simulink model "DA40_Flight_Model"  (R2023a)
settings: Solver=FixedStepAuto  StartTime=DCAM.startTime  StopTime=DCAM.endTime  FixedStep=DCAM.timeStep  RelTol=1e-3
undefined symbols (not defined in the file or in its folder): DCAM, Earth, WGS84
libraries: simulink x27, slpidlib x15, simulink_extras x6, sharedtransform x4, aerolibtransform2 x4, aerolibatmos2 x3, uavalgslib x2, aerolibwind2 x1
(part 5 of 6)

== matlab function DA40_Flight_Model/Correlator Simulation/Subsystem1/Generating GPS and Satellite Measurements/Calculate Satellite Positions/MATLAB Function ==
  data: transmitTime input; satelliteID input; toe input; a_f2 input; a_f1 input; a_f0 input; T_GD input; sqrtA input; Eccentricity input; C_us input; C_uc input; satX output; satY output; satZ output; satU output; satV output; satW output; satClkCorr output; C_rs input; C_rc input; C_is input; C_ic input; M_0 input; iDOT input; i_0 input; OMEGA input; OMEGA_DOT input; delta_n input; OMEGA_0 input
function [satX,satY,satZ,satU,satV,satW,satClkCorr] = satpos(transmitTime,satelliteID,toe,a_f2,a_f1,a_f0,T_GD,sqrtA,Eccentricity,C_us,C_uc,C_rs,C_rc,C_is,C_ic,M_0,iDOT,i_0,OMEGA,OMEGA_DOT,delta_n,OMEGA_0)

%% Initialize constants ===================================================
numOfSatellites = length(satelliteID);

% GPS constatns

gpsPi          = 3.1415926535898;  % Pi used in the GPS coordinate
% system

%--- Constants for satellite position calculation -------------------------
Omegae_dot     = 7.2921151467e-5;  % Earth rotation rate, [rad/s]
GM             = 3.986005e14;      % Earth's universal
% gravitational parameter,
% [m^3/s^2]
F              = -4.442807633e-10; % Constant, [sec/(meter)^(1/2)]

%% Initialize results =====================================================
satClkCorr   = zeros(1,numOfSatellites);
satX = zeros(1,numOfSatellites);
satY = zeros(1,numOfSatellites);
satZ = zeros(1,numOfSatellites);
satU = zeros(1,numOfSatellites);
satV = zeros(1,numOfSatellites);
satW = zeros(1,numOfSatellites);

%% Process each satellite =================================================

for satNr = 1 : numOfSatellites

    %% Find initial satellite clock correction --------------------------------

    %--- Find time difference ---------------------------------------------
    dt = check_t(transmitTime(satNr) - toe(satNr));

    %--- Calculate clock correction ---------------------------------------
    satClkCorr(satNr) = (a_f2(satNr) * dt + a_f1(satNr)) * dt + ...
        a_f0(satNr) - ...
        T_GD(satNr);
    time = transmitTime(satNr) - satClkCorr(satNr);

    %% Find satellite's position ----------------------------------------------

    % Restore semi-major axis
    a   = sqrtA(satNr)*sqrtA(satNr);

    % Time correction
    tk  = check_t(time - toe(satNr));

    % Initial mean motion
    n0  = sqrt(GM/a^3);
    % Mean motion
    n   = n0 + delta_n(satNr);

    % Mean anomaly
    M   = M_0(satNr) + n*tk;
    % Reduce mean anomaly to between 0 and 360 deg
    M   = rem(M + 2*gpsPi, 2*gpsPi);

    % Initial guess of eccentric anomaly
    E   = M;

    %--- Iteratively compute eccentric anomaly ----------------------------
    for ii = 1:10
        E_old   = E;
        E       = M + Eccentricity(satNr) * sin(E);
        dE      = rem(E - E_old, 2*gpsPi);

        if abs(dE) < 1.e-12
            % Necessary precision is reached, exit from the loop
            break;
        end
    end

    % Reduce eccentric anomaly to between 0 and 360 deg
    E   = rem(E + 2*gpsPi, 2*gpsPi);
    dE = n/(1-Eccentricity(satNr) * cos(E));
    % Compute relativistic correction term
    dtr = F * Eccentricity(satNr) * sqrtA(satNr) * sin(E);

    % Calculate the true anomaly
    nu   = atan2(sqrt(1 - Eccentricity(satNr)^2) * sin(E), cos(E)-Eccentricity(satNr));

    %Compute angle phi
    phi = nu + OMEGA(satNr);
    dphi=sqrt(1-Eccentricity(satNr)^2)*dE/(1-Eccentricity(satNr)*cos(E));
    % Reduce phi to between 0 and 360 deg
    phi = rem(phi, 2*gpsPi);

    % Correct argument of latitude
    u = phi + ...
        C_uc(satNr) * cos(2*phi) + ...
        C_us(satNr) * sin(2*phi);
    du=(1+2*(C_us(satNr) * cos(2*phi)-C_uc(satNr) * sin(2*phi)))*dphi;
    % Correct radius
    r = a * (1 - Eccentricity(satNr)*cos(E)) + ...
        C_rc(satNr) * cos(2*phi) + ...
        C_rs(satNr) * sin(2*phi);
    dr= a * Eccentricity(satNr) *sin(E) *dE + ...
        2 * (C_rs(satNr) * cos(2*phi) - C_rc(satNr) * sin(2*phi)) ...
        * dphi;
    % Correct inclination
    i = i_0(satNr) + iDOT(satNr) * tk + ...
        C_ic(satNr) * cos(2*phi) + ...
        C_is(satNr) * sin(2*phi);
    di = 2 * (C_is(satNr) * cos(2*phi) - C_ic(satNr) * sin(2*phi)) ...
        * dphi + iDOT(satNr);

    % Compute the angle between the ascending node and the Greenwich meridian
    Omega = OMEGA_0(satNr) + (OMEGA_DOT(satNr) - Omegae_dot)*tk - ...
        Omegae_dot * toe(satNr);
    dOmega = OMEGA_DOT(satNr) - Omegae_dot;
    % Reduce to between 0 and 360 deg
    Omega = rem(Omega + 2*gpsPi, 2*gpsPi);

    %--- Compute satellite coordinates ------------------------------------
    x = cos(u)*r * cos(Omega) - sin(u)*r * cos(i)*sin(Omega);
    y = cos(u)*r * sin(Omega) + sin(u)*r * cos(i)*cos(Omega);
    z = sin(u)*r * sin(i);

    xdash = r * cos(u);
    ydash = r * sin(u);

    dxdash = dr * cos(u) - r * sin(u) * du;
    dydash = dr * sin(u) + r * cos(u) * du;

    Vx = dxdash * cos(Omega) -  dydash * cos(i) * sin(Omega) ...
        + ydash * sin(Omega) * sin(i) * di - (xdash * sin(Omega) + ...
        ydash * cos(i) * cos(Omega)) * dOmega;

    Vy = dxdash * sin(Omega) + dydash * cos(i) * cos(Omega) - ...
        ydash * sin(i) *cos(Omega) * di + (xdash * cos(Omega) - ...
        ydash * cos(i) * sin(Omega)) * dOmega;

    Vz = dydash * sin(i) + ydash * cos(i) * di;

    satX(satNr) = x;
    satY(satNr) = y;
    satZ(satNr) = z;
    satU(satNr) = Vx;
    satV(satNr) = Vy;
    satW(satNr) = Vz;

    % Include relativistic correction in clock correction --------------------
    satClkCorr(satNr) = (a_f2(satNr) * dt + a_f1(satNr)) * dt + ...
        a_f0(satNr) - ...
        T_GD(satNr) + dtr;

end % for satNr = 1 : numOfSatellites

end

function corrTime = check_t(time)

%CHECKTIME is a subfunction of SATPOS used to check for
%overlapping time in GPS seconds

half_week = 302400;     % seconds

corrTime = time;

if time > half_week
    corrTime = time - 2*half_week;
elseif time < -half_week
    corrTime = time + 2*half_week;
end
end

== matlab function DA40_Flight_Model/Correlator Simulation/Subsystem1/Subsystem2/Generating PSR//Carrier Frequency Measurements/MATLAB Function1 ==
  data: unitVectors input; carrFrequency output; usrU input; usrV input; usrW input; satU input; satV input; satW input; clkDrift input; L1Freq input; IFFreq input
function carrFrequency = calcCarrFreq(unitVectors,usrU,usrV,usrW,satU,satV,satW,clkDrift,L1Freq,IFFreq)

satVel = [satU;satV;satW];
usrVel = [usrU;usrV;usrW];

velLOS = unitVectors.*(satVel - usrVel);
carrFrequency = (1 - velLOS/c)*L1Freq / (1 + clkDrift/c) - L1Freq + IFFreq;

end

== matlab function DA40_Flight_Model/Correlator Simulation/MATLAB Function ==
  data: cno input; pdiTime input; carrFreqError input; codePhaseError input; offset input; IE output; whiteNoise input; QE output; IP output; QP output; IL output; QL output
function [IE,QE,IP,QP,IL,QL] = generateCorrelators(cno,pdiTime,carrFreqError,codePhaseError,offset,whiteNoise)
IE = 0;
QE = 0;
IP = 0;
QP = 0;
IL = 0;
QL = 0;

noise = sqrt(1/cnoL1/pdiTime)*whiteNoise;

IP = sqrt(2*cno*pdiTime)*sinc((carrFreqError)*pdiTime*2*pi)*(1 - abs(codePhaseError))*cos(carrFreqError) + noise(1);
QP = sqrt(2*cno*pdiTime)*sinc((carrFreqError)*pdiTime*2*pi)*(1 - abs(codePhaseError))*sin(carrFreqError) + noise(2);
IE = sqrt(2*cno*pdiTime)*sinc((carrFreqError)*pdiTime*2*pi)*(1 - abs(codePhaseError - offset))*cos(carrFreqError) + noise(3);
QE = sqrt(2*cno*pdiTime)*sinc((carrFreqError)*pdiTime*2*pi)*(1 - abs(codePhaseError - offset))*sin(carrFreqError) + noise(4);
IL = sqrt(2*cno*pdiTime)*sinc((carrFreqError)*pdiTime*2*pi)*(1 - abs(codePhaseError + offset))*cos(carrFreqError) + noise(5);
QL = sqrt(2*cno*pdiTime)*sinc((carrFreqError)*pdiTime*2*pi)*(1 - abs(codePhaseError + offset))*sin(carrFreqError) + noise(6);

end

== matlab function DA40_Flight_Model/Correlator Simulation/Subsystem1/Generating GPS and Satellite Measurements/Truth Model/Navigation1/Flight Mechanics and Systems Models/Engine + Prop Model/Subsystem/Air Flow Rate Exam 1 ==
  data: Tatm_K input; Pman_inHg input; throttle input; Patm_inHg input; Air_lb_hr output
function Air_lb_hr  = Calc_Air_Flow(Tatm_K,Pman_inHg,throttle,Patm_inHg)
%% Conversion Factors
inHg_to_Pa = 3386.39;
in2_to_m2 = 0.00064516;
kg_to_lb = 2.20462;
%% Constants
gamma = 1.4;
R = 287;
AirflowScaler = 0.69 * 0.95;
DischargeCoeff = 0.6;
th = 70*throttle;
D = 2.75;

Patm_Pa = Patm_inHg * inHg_to_Pa;
Pman_Pa = Pman_inHg * inHg_to_Pa;
A_in2 = (pi/4) * D^2 *  (0.01 + (1-0.01)*(1 - cosd(th)));
A_m2 = A_in2 * in2_to_m2;

Threshold_X = (2/(gamma+1))^(gamma/(gamma-1));

x = Threshold_X;

MAF = sqrt((2*gamma/(gamma-1))*(x^(2/gamma)-x^((gamma+1)/gamma)));

MassFlux_kgm2s = MAF*Patm_Pa/sqrt(R*Tatm_K);
MassFlow_kgs = MassFlux_kgm2s * A_m2; 

Air_lb_hr = AirflowScaler*DischargeCoeff*MassFlow_kgs*3600*kg_to_lb;
end

== matlab function DA40_Flight_Model/Correlator Simulation/Subsystem1/Generating GPS and Satellite Measurements/Truth Model/Navigation1/Flight Mechanics and Systems Models/Engine + Prop Model/Subsystem/Engine Shaft Power and Torque Model ==
  data: wdot_f input; PF input; BSFC input; P_shaft output
function P_shaft  = fcn(wdot_f,PF,BSFC)

P_shaft = PF*wdot_f/BSFC; %hp

% Q_drive = P_shaft*746/Omega; %Nm


end

== matlab function DA40_Flight_Model/Correlator Simulation/Subsystem1/Generating GPS and Satellite Measurements/Truth Model/Navigation1/Flight Mechanics and Systems Models/Engine + Prop Model/Subsystem/MATLAB Function ==
  data: X input; Aircraft_Airspeed output
function Aircraft_Airspeed = Calc_AC_Speed(X)
Aircraft_Airspeed = norm(X(1:3));
end

== matlab function DA40_Flight_Model/Correlator Simulation/Subsystem1/Generating GPS and Satellite Measurements/Truth Model/Navigation1/Flight Mechanics and Systems Models/Engine + Prop Model/Subsystem/Manifold Pressure Calculation ==
  data: throttle input; Patm_inHg input; N input; Pman_inHg output; throttle output; Patm_inHg output
function [Pman_inHg,throttle,Patm_inHg]  = fcn(throttle,Patm_inHg,N)

Pman_inHg = Patm_inHg + (0.007*throttle - 0.0086)*N;

end

== matlab function DA40_Flight_Model/Correlator Simulation/Subsystem1/Generating GPS and Satellite Measurements/Truth Model/Navigation1/Flight Mechanics and Systems Models/Engine + Prop Model/Subsystem/Propeller Dynamics ==
  data: V input; power input; Q_drive input size=1; Prop_Pitch input; rho input; n input; T output; Q output; eta_p output size=1; dOmega_dt output
function [T,Q,eta_p,dOmega_dt] = VarP_PropDynamics(V,power, Q_drive,Prop_Pitch,rho,n)

T = 0;
Q = 0;
eta_p = 0;
dOmega_dt = 0;

coder.extrinsic('griddedInterpolant')
coder.extrinsic('CTCQPropeff')

[T,Q,eta_p,dOmega_dt] = CTCQPropeff(Prop_Pitch,power,Q_drive,rho,V,n,[]);

end

== matlab function DA40_Flight_Model/Correlator Simulation/Subsystem1/Generating GPS and Satellite Measurements/Truth Model/Navigation1/Flight Mechanics and Systems Models/Gear/  ==
  data: U input; X input; mu input; Ground_Forces output; Ground_Moments output
function [Ground_Forces,Ground_Moments] = LDG_Model(U,X,mu)
%% Ground Contact points taken from powerpoint
Front_LDG = [1.634;0;0.983]';
Right_MG = [-0.5;1.447;0.893]';
Left_MG = [-0.5;-1.447;0.893]';
Prop_Strike = [2.379;0;0.847]';
Right_Wing = [0;5.53;-0.087]';
Left_Wing = [0;-5.53;-0.087]';
Tail_Strike = [-4.552;0;0.271]';
GC = [Front_LDG;Right_MG;Left_MG;Prop_Strike;Right_Wing;Left_Wing;Tail_Strike];
%% Spring and Damper Coeffs
k_r = 80000;
c_r = 14300;

k_f = 50000;
c_f = 11300;

k_b = 280000;
c_b = 26800;
%% Defining State Vector to make the coding easier
u = X(1);
v = X(2);
w = X(3);
p = X(4);
q = X(5);
r = X(6);
x = X(7);
y = X(8);
z = X(9);
phi = X(10);
theta = X(11);
psi = X(12);

ALTdot = -w;
ALT = -z;
%% State Derivatives
phidot = p + q*sin(phi)*tan(theta) + r*cos(phi)*tan(theta);
thetadot = q*cos(phi) - r*sin(phi);
%% Controls from Pilot
Brake_Setting = (U(1) + U(2))/2;
Steering_Control = U(3);
%% Friction while plane is in motion
Rolling_Friction = mu(1);
%% Calculations
%% Have to calculate each components distance from the ground...
del_S = zeros(7,1);
del_S_dot = zeros(7,1);
F = zeros(7,3);

del_S(1) = ALT + Front_LDG(1)*sin(theta) - Front_LDG(2)*sin(phi)*cos(theta) - Front_LDG(3)*cos(phi)*cos(theta);
del_S(2) = ALT + Right_MG(1)*sin(theta) - Right_MG(2)*sin(phi)*cos(theta) - Right_MG(3)*cos(phi)*cos(theta);
del_S(3) = ALT + Left_MG(1)*sin(theta) - Left_MG(2)*sin(phi)*cos(theta) - Left_MG(3)*cos(phi)*cos(theta);
del_S(4) = ALT + Prop_Strike(1)*sin(theta) - Prop_Strike(2)*sin(phi)*cos(theta) - Prop_Strike(3)*cos(phi)*cos(theta);
del_S(5) = ALT + Right_Wing(1)*sin(theta) - Right_Wing(2)*sin(phi)*cos(theta) - Right_Wing(3)*cos(phi)*cos(theta);
del_S(6) = ALT + Left_Wing(1)*sin(theta) - Left_Wing(2)*sin(phi)*cos(theta) - Left_Wing(3)*cos(phi)*cos(theta);
del_S(7) = ALT + Tail_Strike(1)*sin(theta) - Tail_Strike(2)*sin(phi)*cos(theta) - Tail_Strike(3)*cos(phi)*cos(theta);

%deltaS order
% 1 Nose Gear
% 2 Right Main Gear
% 3 Left Main Gear
% 4 Prop Strike
% 5 Right Wingtip
% 6 Left Wingtip
% 7 Tail Strike

del_S_dot(1) = ALTdot + Front_LDG(1)*cos(theta)*thetadot + Front_LDG(2)*(thetadot*sin(phi)*sin(theta) - phidot*cos(phi)*cos(theta)) + Front_LDG(3)*(thetadot*sin(theta)*cos(phi) + phidot*sin(theta)*sin(phi))+ del_S(1)*(cos(phi)*sin(theta)*thetadot + sin(phi)*cos(theta)*phidot);
if del_S(1) < 0
    F(1,3) = k_f*del_S(1) + c_f*del_S_dot(1);
else
    F(1,3) = 0;
end
del_S_dot(2) = ALTdot + Right_MG(1)*cos(theta)*thetadot + Right_MG(2)*(thetadot*sin(phi)*sin(theta) - phidot*cos(phi)*cos(theta)) + Right_MG(3)*(thetadot*sin(theta)*cos(phi) + phidot*sin(theta)*sin(phi))+ del_S(2)*(cos(phi)*sin(theta)*thetadot + sin(phi)*cos(theta)*phidot);
if del_S(2) < 0
    F(2,3) = k_r*del_S(2) + c_r*del_S_dot(2);
else
    F(2,3) = 0;
end
del_S_dot(3) = ALTdot + Left_MG(1)*cos(theta)*thetadot + Left_MG(2)*(thetadot*sin(phi)*sin(theta) - phidot*cos(phi)*cos(theta)) + Left_MG(3)*(thetadot*sin(theta)*cos(phi) + phidot*sin(theta)*sin(phi))+ del_S(3)*(cos(phi)*sin(theta)*thetadot + sin(phi)*cos(theta)*phidot);
if del_S(3) < 0
    F(3,3) = k_r*del_S(3) + c_r*del_S_dot(3);
else
    F(3,3) = 0;
end
del_S_dot(4) = ALTdot + Prop_Strike(1)*cos(theta)*thetadot + Prop_Strike(2)*(thetadot*sin(phi)*sin(theta) - phidot*cos(phi)*cos(theta)) + Prop_Strike(3)*(thetadot*sin(theta)*cos(phi) + phidot*sin(theta)*sin(phi));
if del_S(4) < 0
    F(4,3) = k_b*del_S(4) + c_b*del_S_dot(4);
else
    F(4,3) = 0;
end
del_S_dot(5) = ALTdot + Right_Wing(1)*cos(theta)*thetadot + Right_Wing(2)*(thetadot*sin(phi)*sin(theta) - phidot*cos(phi)*cos(theta)) + Right_Wing(3)*(thetadot*sin(theta)*cos(phi) + phidot*sin(theta)*sin(phi));
if del_S(5) < 0
    F(5,3) = k_b*del_S(5) + c_b*del_S_dot(5);
else
    F(5,3) = 0;
end
del_S_dot(6) = ALTdot + Left_Wing(1)*cos(theta)*thetadot + Left_Wing(2)*(thetadot*sin(phi)*sin(theta) - phidot*cos(phi)*cos(theta))+ Left_Wing(3)*(thetadot*sin(theta)*cos(phi) + phidot*sin(theta)*sin(phi));
if del_S(6) < 0
    F(6,3) = k_b*del_S(6) + c_b*del_S_dot(6);
else
    F(6,3) = 0;
end

del_S_dot(7) = ALTdot + Tail_Strike(1)*cos(theta)*thetadot + Tail_Strike(2)*(thetadot*sin(phi)*sin(theta) - phidot*cos(phi)*cos(theta)) + Tail_Strike(3)*(thetadot*sin(theta)*cos(phi) + phidot*sin(theta)*sin(phi));
if del_S(7) < 0
    F(7,3) = k_b*del_S(7) + c_b*del_S_dot(7);
else
    F(7,3) = 0;
end
%% Calculating the velo seen by the LDG

VxB = u - r.*GC(:,2) + q.*(GC(:,3) + del_S);
VyB = v + r.*GC(:,1) - p.*(GC(:,3) + del_S);
VzB = w - q.*GC(:,1) + p.*GC(:,2);

Vxge = cos(theta).*VxB + (sin(phi).*sin(theta)).*VyB + (cos(phi)*sin(theta)).*VzB;
Vyge = cos(phi).*VyB + (-sin(phi)).*VzB;

Steering_Control = [Steering_Control,0,0,0,0,0,0]';
uk  = VxB.*cos(Steering_Control) + VyB.*sin(Steering_Control);

mu_s = 0.8;
C_p = 1.1;
B_p = 7;
mu_br = 0.7*Brake_Setting;
mu_rb = zeros(3,1);
mu_Y = zeros(3,1);
for i = 1:3
    if abs(uk(i)) < 1e-4
        mu_rb(i) = 0;
    else
        mu_rb(i) =  (Rolling_Friction + mu_br).*sign(uk(i));
    end
    
    mu_y_max = sqrt(mu_s^2 - mu_rb(i)^2);
    Sy =  Steering_Control(i) - atan(Vyge(i)/(Vxge(i) + 0.00000001 ));
    if abs(uk(i)) < 0.001
        mu_Y(i) = 0;
    else
        mu_Y(i) = -mu_y_max*sin(C_p*atan(B_p.*Sy));
    end
end
%% Calculating the x and y forces...
F(1:3,1) = mu_rb.*F(1:3,3);
F(1:3,2) = mu_Y.*F(1:3,3);
%% Converting to Body-Fixed Axis to output...
F_B = zeros(7,3);
F_B(:,1) = cos(theta).*cos(-Steering_Control).*F(:,1) + cos(theta).*F(:,2) - sin(theta).*F(:,3);
F_B(:,2)= (sin(phi).*sin(theta).*cos(-Steering_Control)-cos(phi).*sin(-Steering_Control)).*F(:,1) + (sin(phi).*sin(theta).*sin(-Steering_Control) + cos(phi).*cos(-Steering_Control)).*F(:,2) + sin(phi).*cos(theta).*F(:,3);
F_B(:,3) = (cos(phi).*sin(theta).*cos(-Steering_Control) + sin(phi).*sin(-Steering_Control)).*F(:,1) + (cos(phi).*sin(theta).*sin(-Steering_Control)-sin(phi).*cos(-Steering_Control)).*F(:,2) + (cos(phi).*cos(theta)).*F(:,3);

NG_Mom = cross(Front_LDG,F(1,:));
RMG_Mom = cross(Right_MG, F(2,:));
LMG_Mom = cross(Left_MG, F(3,:));
Prop_Strike_Mom = cross(Prop_Strike,F(4,:));
RWT_Mom = cross(Right_Wing,F(5,:));
LWT_Mom = cross(Left_Wing,F(6,:));
Tail_Strike_Mom = cross(Tail_Strike, F(7,:));

Ground_Forces = [sum(F_B(:,1)),sum(F_B(:,2)),sum(F_B(:,3))];
Ground_Moments = (NG_Mom + RMG_Mom + LMG_Mom + Prop_Strike_Mom + RWT_Mom + LWT_Mom + Tail_Strike_Mom);
end

== matlab function DA40_Flight_Model/Correlator Simulation/Subsystem1/Generating GPS and Satellite Measurements/Truth Model/Navigation1/Flight Mechanics and Systems Models/Gravity/MATLAB Function ==
  data: X input; F_grav_b output; Mass_Properties input; CG input; M_grav_b output
function [F_grav_b,M_grav_b] = Grav_Forces(X,Mass_Properties,CG)
%% Defining State Vector to Code Easier
u = X(1);
v = X(2);
w = X(3);
p = X(4);
q = X(5);
r = X(6);
x = X(7);
y = X(8);
z = X(9);
phi = X(10);
theta = X(11);
psi = X(12);

g = 9.81;

F_grav_b = Mass_Properties.*[-g*sin(theta);g*sin(phi)*cos(theta);g*cos(phi)*cos(theta)];

M_grav_b = cross(CG,F_grav_b);

== matlab function DA40_Flight_Model/Correlator Simulation/Subsystem1/Generating GPS and Satellite Measurements/Truth Model/Navigation1/Flight Mechanics and Systems Models/Strip Theory Aero + Propulsive Forces/Strip_Theory_Modeling ==
  data: atmos input; X input; U input; stripGeom input; Strip_Theory_Forces output; Strip_Theory_Moments output
function [Strip_Theory_Forces,Strip_Theory_Moments] = Strip_Theory(atmos,X,U,stripGeom)
Strip_Theory_Forces = [0;0;0];
Strip_Theory_Moments = [0;0;0];

coder.extrinsic('griddedInterpolant')
coder.extrinsic('AC_Strip_Theory')

[Strip_Theory_Forces,Strip_Theory_Moments] = AC_Strip_Theory(atmos(4),X,U,stripGeom);

== matlab function DA40_Flight_Model/Correlator Simulation/Subsystem/MATLAB Function1 ==
  data: measuredCarrierFrequency input; carrFreqError output; estimatedCarrierFrequency input
function carrFreqError = calcCarrierFrequencyError(measuredCarrierFrequency,estimatedCarrierFrequency)

carrFreqError = mean(measuredCarrierFrequency - estimatedCarrierFrequency);

end

== matlab function DA40_Flight_Model/Correlator Simulation/Subsystem/MATLAB Function2 ==
  data: measuredCodeFrequency input; codeFreqError output; estimatedCodeFrequency input
function codeFreqError = calcCarrierFrequencyError(measuredCodeFrequency,estimatedCodeFrequency)

codeFreqError = measuredCodeFrequency - estimatedCodeFrequency;

end

== matlab function DA40_Flight_Model/Correlator Simulation/Subsystem1/Subsystem2/Subsystem1/MATLAB Function3 ==
  data: sampleVector input; MeasuredCarrierFrequency output; carrierChangePerSample input; measuredCarrierFrequency input
function MeasuredCarrierFrequency = calcMeasuredCarrierFrequency(sampleVector,carrierChangePerSample,measuredCarrierFrequency)

MeasuredCarrierFrequency = sampleVector*carrierChangePerSample + measuredCarrierFrequency;

end

== matlab function DA40_Flight_Model/Correlator Simulation/Subsystem1/Subsystem2/Subsystem3/Subsystem2/MATLAB Function4 ==
  data: samplesPerPDI input; initialCarrierFrequency input; sampleVector output; carrierChangePerSample output; measuredCarrierFrequency input
function [sampleVector,carrierChangePerSample]  = fcn(samplesPerPDI,initialCarrierFrequency,measuredCarrierFrequency)

sampleVector = 0:samplesPerPDI;
carrierChangePerSample = (measuredCarrierFrequency - initialCarrierFrequency)/samplesPerPDI;

end

== matlab function DA40_Flight_Model/Correlator Simulation/Subsystem1/Subsystem2/Generating PSR//Carrier Frequency Measurements2/MATLAB Function ==
  data: usrX input; usrY input; usrZ input; clk input; pseudoranges output; satX input; satY input; satZ input; unitVectors output
function [pseudoranges,unitVectors] = calcPSR(usrX,usrY,usrZ,clk,satX,satY,satZ)

dx2 = (usrX - satX).^2;
dy2 = (usrY - satY).^2;
dz2 = (usrZ - satZ).^2;

r = sqrt(dx2 + dy2 + dz2);
pseudoranges =  r + clk;

ux = (usrX - satX)./r;
uy = (usrY - satY)./r;
uz = (usrZ - satZ)./r;

unitVectors = [ux;uy;uz];

end

== matlab function DA40_Flight_Model/Extended Kalman Filter/Noise Model/Environment/MATLAB Function7 ==
  data: RotAngles input; DCM output; RotSequence input
function DCM = MyDCMFunction(RotAngles,RotSequence)
n = length(RotSequence);
Matrix = zeros(3,3,3);
for i = 1:n
    k = RotSequence(i);
    switch k
        case 1
            Matrix(:,:,i) = [1 0 0;0 cosd(RotAngles(i)) -sind(RotAngles(i));0 sind(RotAngles(i)) cosd(RotAngles(i))];
        case 2
            Matrix(:,:,i) = [cosd(RotAngles(i)) 0 sind(RotAngles(i));0 1 0;-sind(RotAngles(i)) 0 cosd(RotAngles(i))];
        case 3
            Matrix(:,:,i) = [cosd(RotAngles(i)) -sind(RotAngles(i)) 0;sind(RotAngles(i)) cosd(RotAngles(i)) 0;0 0 1];
    end
end
p = 1;
while p < n
    Matrix(:,:,p+1) = Matrix(:,:,p) * Matrix(:,:,p+1);
    p = p + 1;
end
DCM = Matrix(:,:,p);
end

== matlab function DA40_Flight_Model/Correlator Simulation/Subsystem1/Subsystem2/Generating PSR//Carrier Frequency Measurements2/MATLAB Function1 ==
  data: unitVectors input; carrFrequency output; usrU input; usrV input; usrW input; satU input; satV input; satW input; clkDrift input; L1Freq input; IFFreq input
function carrFrequency = calcCarrFreq(unitVectors,usrU,usrV,usrW,satU,satV,satW,clkDrift,L1Freq,IFFreq)

satVel = [satU;satV;satW];
usrVel = [usrU;usrV;usrW];

velLOS = unitVectors.*(satVel - usrVel);
carrFrequency = (1 - velLOS/c)*L1Freq / (1 + clkDrift/c) - L1Freq + IFFreq;

end

== matlab function DA40_Flight_Model/Correlator Simulation/Subsystem1/Subsystem2/Subsystem1/MATLAB Function1 ==
  data: sampleVector input; MeasuredCodeFrequency output; codeChangePerSample input; initialCodePhase input
function MeasuredCodeFrequency = calcMeasuredCodeFrequency(sampleVector,codeChangePerSample,initialCodePhase)

MeasuredCodeFrequency = sampleVector*codeChangePerSample + measuredCarrierFrequency;

trueCodePhase = sampleVec(idx)*codeChangePerSample + initialCodePhase;
trueCodePhase = trueCodePhaseVec(idx);

end

== matlab function DA40_Flight_Model/Correlator Simulation/Subsystem1/Generating GPS and Satellite Measurements/Truth Model/Control/Subsystem3/MATLAB Function ==
  data: X input; Aircraft_Airspeed output
function Aircraft_Airspeed = Calc_AC_Speed(X)
Aircraft_Airspeed = norm(X(1:3));
end

== matlab function DA40_Flight_Model/Extended Kalman Filter/Noise Model/Navigation/DA-40 Equations of Motion/MATLAB Function4 ==
  data: m input; X_Dot output size=12; Ic_B input; F_B input; M_B input; X input; CG input; InvMassMatrix input
function X_Dot  = CalcXdot(m,Ic_B,F_B,M_B,X,CG,InvMassMatrix)
X_Dot = zeros(12,1);
% muVector = zeros(3,1);
u = X(1);
v = X(2);
w = X(3);
p = X(4);
q = X(5);
r = X(6);
x = X(7);
y = X(8);
z = X(9);
phi = X(10);
theta = X(11);
psi = X(12);


Xcg = CG(1);
Ycg = CG(2);
Zcg = CG(3);

CGssm = [0 -Zcg Ycg;Zcg 0 -Xcg;-Ycg Xcg 0];


lambdaX = F_B(1)/m + r*v - q*w - 0 - 2*q*0 + 2*r*0 + Xcg*(q^2 + r^2) - Ycg*p*q - Zcg*p*r;
lambdaY = F_B(2)/m + p*w - r*u - 0 - 2*r*0 + 2*p*0 - Xcg*p*q + Ycg*(p^2 +r^2) - Zcg*q*r;
lambdaZ = F_B(3)/m + q*u - p*v - 0 - 2*p*0 + 2*q*0 - Xcg*p*r - Ycg*q*r + Zcg*(p^2 + q^2);

MomentVector = [p;q;r];

MomentVectorssm = [0 -r q;r 0 -p;-q p 0];

muVector = [M_B(1);M_B(2);M_B(3)] - (MomentVectorssm*Ic_B*MomentVector) - m*CGssm*MomentVectorssm*[u;v;w];
LAMEparams = [lambdaX;lambdaY;lambdaZ;muVector];
X_Dot(1:6) = InvMassMatrix*LAMEparams;

cphi = cos(phi);
sphi = sin(phi);

ctheta = cos(theta);
stheta = sin(theta);
ttheta = tan(theta);

cpsi = cos(psi);
spsi = sin(psi);

xdot = ctheta*cpsi*u + sphi*stheta*cpsi - cphi*spsi*v + cphi*stheta*cpsi + sphi*spsi*w;
ydot = ctheta*spsi*u + sphi*stheta*spsi + cphi*cpsi*v + cphi*stheta*spsi - sphi*cpsi*w;
zdot = -stheta*u + sphi*ctheta*v + cphi*ctheta*w;
phidot = p + q*sphi*ttheta + r*cphi*ttheta;
thdot = q*cphi - r*sphi;
psidot = q*sphi/ctheta + r*cphi/ctheta;
X_Dot(7:12) = [xdot;ydot;zdot;phidot;thdot;psidot];

end

== matlab function DA40_Flight_Model/Extended Kalman Filter/Noise Model/Navigation/Flight Mechanics and Systems Models/Engine + Prop Model/Subsystem/Air Flow Rate Exam 1 ==
  data: Tatm_K input; Pman_inHg input; throttle input; Patm_inHg input; Air_lb_hr output
function Air_lb_hr  = Calc_Air_Flow(Tatm_K,Pman_inHg,throttle,Patm_inHg)
%% Conversion Factors
inHg_to_Pa = 3386.39;
in2_to_m2 = 0.00064516;
kg_to_lb = 2.20462;
%% Constants
gamma = 1.4;
R = 287;
AirflowScaler = 0.69 * 0.95;
DischargeCoeff = 0.6;
th = 70*throttle;
D = 2.75;

Patm_Pa = Patm_inHg * inHg_to_Pa;
Pman_Pa = Pman_inHg * inHg_to_Pa;
A_in2 = (pi/4) * D^2 *  (0.01 + (1-0.01)*(1 - cosd(th)));
A_m2 = A_in2 * in2_to_m2;

Threshold_X = (2/(gamma+1))^(gamma/(gamma-1));

x = Threshold_X;

MAF = sqrt((2*gamma/(gamma-1))*(x^(2/gamma)-x^((gamma+1)/gamma)));

MassFlux_kgm2s = MAF*Patm_Pa/sqrt(R*Tatm_K);
MassFlow_kgs = MassFlux_kgm2s * A_m2; 

Air_lb_hr = AirflowScaler*DischargeCoeff*MassFlow_kgs*3600*kg_to_lb;
end

== matlab function DA40_Flight_Model/Extended Kalman Filter/Noise Model/Navigation/Flight Mechanics and Systems Models/Engine + Prop Model/Subsystem/Engine Shaft Power and Torque Model ==
  data: wdot_f input; PF input; BSFC input; P_shaft output
function P_shaft  = fcn(wdot_f,PF,BSFC)

P_shaft = PF*wdot_f/BSFC; %hp

% Q_drive = P_shaft*746/Omega; %Nm


end

== matlab function DA40_Flight_Model/Extended Kalman Filter/Noise Model/Navigation/Flight Mechanics and Systems Models/Engine + Prop Model/Subsystem/MATLAB Function ==
  data: X input; Aircraft_Airspeed output
function Aircraft_Airspeed = Calc_AC_Speed(X)
Aircraft_Airspeed = norm(X(1:3));
end

== matlab function DA40_Flight_Model/Extended Kalman Filter/Noise Model/Navigation/Flight Mechanics and Systems Models/Engine + Prop Model/Subsystem/Manifold Pressure Calculation ==
  data: throttle input; Patm_inHg input; N input; Pman_inHg output; throttle output; Patm_inHg output
function [Pman_inHg,throttle,Patm_inHg]  = fcn(throttle,Patm_inHg,N)

Pman_inHg = Patm_inHg + (0.007*throttle - 0.0086)*N;

end

== matlab function DA40_Flight_Model/Extended Kalman Filter/Noise Model/Navigation/Flight Mechanics and Systems Models/Engine + Prop Model/Subsystem/Propeller Dynamics ==
  data: V input; power input; Q_drive input size=1; Prop_Pitch input; rho input; n input; T output; Q output; eta_p output size=1; dOmega_dt output
function [T,Q,eta_p,dOmega_dt] = VarP_PropDynamics(V,power, Q_drive,Prop_Pitch,rho,n)

T = 0;
Q = 0;
eta_p = 0;
dOmega_dt = 0;

coder.extrinsic('griddedInterpolant')
coder.extrinsic('CTCQPropeff')

[T,Q,eta_p,dOmega_dt] = CTCQPropeff(Prop_Pitch,power,Q_drive,rho,V,n,[]);

end

== matlab function DA40_Flight_Model/Extended Kalman Filter/Noise Model/Navigation/Flight Mechanics and Systems Models/Gear/  ==
  data: U input; X input; mu input; Ground_Forces output; Ground_Moments output
function [Ground_Forces,Ground_Moments] = LDG_Model(U,X,mu)
%% Ground Contact points taken from powerpoint
Front_LDG = [1.634;0;0.983]';
Right_MG = [-0.5;1.447;0.893]';
Left_MG = [-0.5;-1.447;0.893]';
Prop_Strike = [2.379;0;0.847]';
Right_Wing = [0;5.53;-0.087]';
Left_Wing = [0;-5.53;-0.087]';
Tail_Strike = [-4.552;0;0.271]';
GC = [Front_LDG;Right_MG;Left_MG;Prop_Strike;Right_Wing;Left_Wing;Tail_Strike];
%% Spring and Damper Coeffs
k_r = 80000;
c_r = 14300;

k_f = 50000;
c_f = 11300;

k_b = 280000;
c_b = 26800;
%% Defining State Vector to make the coding easier
u = X(1);
v = X(2);
w = X(3);
p = X(4);
q = X(5);
r = X(6);
x = X(7);
y = X(8);
z = X(9);
phi = X(10);
theta = X(11);
psi = X(12);

ALTdot = -w;
ALT = -z;
%% State Derivatives
phidot = p + q*sin(phi)*tan(theta) + r*cos(phi)*tan(theta);
thetadot = q*cos(phi) - r*sin(phi);
%% Controls from Pilot
Brake_Setting = (U(1) + U(2))/2;
Steering_Control = U(3);
%% Friction while plane is in motion
Rolling_Friction = mu(1);
%% Calculations
%% Have to calculate each components distance from the ground...
del_S = zeros(7,1);
del_S_dot = zeros(7,1);
F = zeros(7,3);

del_S(1) = ALT + Front_LDG(1)*sin(theta) - Front_LDG(2)*sin(phi)*cos(theta) - Front_LDG(3)*cos(phi)*cos(theta);
del_S(2) = ALT + Right_MG(1)*sin(theta) - Right_MG(2)*sin(phi)*cos(theta) - Right_MG(3)*cos(phi)*cos(theta);
del_S(3) = ALT + Left_MG(1)*sin(theta) - Left_MG(2)*sin(phi)*cos(theta) - Left_MG(3)*cos(phi)*cos(theta);
del_S(4) = ALT + Prop_Strike(1)*sin(theta) - Prop_Strike(2)*sin(phi)*cos(theta) - Prop_Strike(3)*cos(phi)*cos(theta);
del_S(5) = ALT + Right_Wing(1)*sin(theta) - Right_Wing(2)*sin(phi)*cos(theta) - Right_Wing(3)*cos(phi)*cos(theta);
del_S(6) = ALT + Left_Wing(1)*sin(theta) - Left_Wing(2)*sin(phi)*cos(theta) - Left_Wing(3)*cos(phi)*cos(theta);
del_S(7) = ALT + Tail_Strike(1)*sin(theta) - Tail_Strike(2)*sin(phi)*cos(theta) - Tail_Strike(3)*cos(phi)*cos(theta);

%deltaS order
% 1 Nose Gear
% 2 Right Main Gear
% 3 Left Main Gear
% 4 Prop Strike
% 5 Right Wingtip
% 6 Left Wingtip
% 7 Tail Strike

del_S_dot(1) = ALTdot + Front_LDG(1)*cos(theta)*thetadot + Front_LDG(2)*(thetadot*sin(phi)*sin(theta) - phidot*cos(phi)*cos(theta)) + Front_LDG(3)*(thetadot*sin(theta)*cos(phi) + phidot*sin(theta)*sin(phi))+ del_S(1)*(cos(phi)*sin(theta)*thetadot + sin(phi)*cos(theta)*phidot);
if del_S(1) < 0
    F(1,3) = k_f*del_S(1) + c_f*del_S_dot(1);
else
    F(1,3) = 0;
end
del_S_dot(2) = ALTdot + Right_MG(1)*cos(theta)*thetadot + Right_MG(2)*(thetadot*sin(phi)*sin(theta) - phidot*cos(phi)*cos(theta)) + Right_MG(3)*(thetadot*sin(theta)*cos(phi) + phidot*sin(theta)*sin(phi))+ del_S(2)*(cos(phi)*sin(theta)*thetadot + sin(phi)*cos(theta)*phidot);
if del_S(2) < 0
    F(2,3) = k_r*del_S(2) + c_r*del_S_dot(2);
else
    F(2,3) = 0;
end
del_S_dot(3) = ALTdot + Left_MG(1)*cos(theta)*thetadot + Left_MG(2)*(thetadot*sin(phi)*sin(theta) - phidot*cos(phi)*cos(theta)) + Left_MG(3)*(thetadot*sin(theta)*cos(phi) + phidot*sin(theta)*sin(phi))+ del_S(3)*(cos(phi)*sin(theta)*thetadot + sin(phi)*cos(theta)*phidot);
if del_S(3) < 0
    F(3,3) = k_r*del_S(3) + c_r*del_S_dot(3);
else
    F(3,3) = 0;
end
del_S_dot(4) = ALTdot + Prop_Strike(1)*cos(theta)*thetadot + Prop_Strike(2)*(thetadot*sin(phi)*sin(theta) - phidot*cos(phi)*cos(theta)) + Prop_Strike(3)*(thetadot*sin(theta)*cos(phi) + phidot*sin(theta)*sin(phi));
if del_S(4) < 0
    F(4,3) = k_b*del_S(4) + c_b*del_S_dot(4);
else
    F(4,3) = 0;
end
del_S_dot(5) = ALTdot + Right_Wing(1)*cos(theta)*thetadot + Right_Wing(2)*(thetadot*sin(phi)*sin(theta) - phidot*cos(phi)*cos(theta)) + Right_Wing(3)*(thetadot*sin(theta)*cos(phi) + phidot*sin(theta)*sin(phi));
if del_S(5) < 0
    F(5,3) = k_b*del_S(5) + c_b*del_S_dot(5);
else
    F(5,3) = 0;
end
del_S_dot(6) = ALTdot + Left_Wing(1)*cos(theta)*thetadot + Left_Wing(2)*(thetadot*sin(phi)*sin(theta) - phidot*cos(phi)*cos(theta))+ Left_Wing(3)*(thetadot*sin(theta)*cos(phi) + phidot*sin(theta)*sin(phi));
if del_S(6) < 0
    F(6,3) = k_b*del_S(6) + c_b*del_S_dot(6);
else
    F(6,3) = 0;
end

del_S_dot(7) = ALTdot + Tail_Strike(1)*cos(theta)*thetadot + Tail_Strike(2)*(thetadot*sin(phi)*sin(theta) - phidot*cos(phi)*cos(theta)) + Tail_Strike(3)*(thetadot*sin(theta)*cos(phi) + phidot*sin(theta)*sin(phi));
if del_S(7) < 0
    F(7,3) = k_b*del_S(7) + c_b*del_S_dot(7);
else
    F(7,3) = 0;
end
%% Calculating the velo seen by the LDG

VxB = u - r.*GC(:,2) + q.*(GC(:,3) + del_S);
VyB = v + r.*GC(:,1) - p.*(GC(:,3) + del_S);
VzB = w - q.*GC(:,1) + p.*GC(:,2);

Vxge = cos(theta).*VxB + (sin(phi).*sin(theta)).*VyB + (cos(phi)*sin(theta)).*VzB;
Vyge = cos(phi).*VyB + (-sin(phi)).*VzB;

Steering_Control = [Steering_Control,0,0,0,0,0,0]';
uk  = VxB.*cos(Steering_Control) + VyB.*sin(Steering_Control);

mu_s = 0.8;
C_p = 1.1;
B_p = 7;
mu_br = 0.7*Brake_Setting;
mu_rb = zeros(3,1);
mu_Y = zeros(3,1);
for i = 1:3
    if abs(uk(i)) < 1e-4
        mu_rb(i) = 0;
    else
        mu_rb(i) =  (Rolling_Friction + mu_br).*sign(uk(i));
    end
    
    mu_y_max = sqrt(mu_s^2 - mu_rb(i)^2);
    Sy =  Steering_Control(i) - atan(Vyge(i)/(Vxge(i) + 0.00000001 ));
    if abs(uk(i)) < 0.001
        mu_Y(i) = 0;
    else
        mu_Y(i) = -mu_y_max*sin(C_p*atan(B_p.*Sy));
    end
end
%% Calculating the x and y forces...
F(1:3,1) = mu_rb.*F(1:3,3);
F(1:3,2) = mu_Y.*F(1:3,3);
%% Converting to Body-Fixed Axis to output...
F_B = zeros(7,3);
F_B(:,1) = cos(theta).*cos(-Steering_Control).*F(:,1) + cos(theta).*F(:,2) - sin(theta).*F(:,3);
F_B(:,2)= (sin(phi).*sin(theta).*cos(-Steering_Control)-cos(phi).*sin(-Steering_Control)).*F(:,1) + (sin(phi).*sin(theta).*sin(-Steering_Control) + cos(phi).*cos(-Steering_Control)).*F(:,2) + sin(phi).*cos(theta).*F(:,3);
F_B(:,3) = (cos(phi).*sin(theta).*cos(-Steering_Control) + sin(phi).*sin(-Steering_Control)).*F(:,1) + (cos(phi).*sin(theta).*sin(-Steering_Control)-sin(phi).*cos(-Steering_Control)).*F(:,2) + (cos(phi).*cos(theta)).*F(:,3);

NG_Mom = cross(Front_LDG,F(1,:));
RMG_Mom = cross(Right_MG, F(2,:));
LMG_Mom = cross(Left_MG, F(3,:));
Prop_Strike_Mom = cross(Prop_Strike,F(4,:));
RWT_Mom = cross(Right_Wing,F(5,:));
LWT_Mom = cross(Left_Wing,F(6,:));
Tail_Strike_Mom = cross(Tail_Strike, F(7,:));

Ground_Forces = [sum(F_B(:,1)),sum(F_B(:,2)),sum(F_B(:,3))];
Ground_Moments = (NG_Mom + RMG_Mom + LMG_Mom + Prop_Strike_Mom + RWT_Mom + LWT_Mom + Tail_Strike_Mom);
end

== matlab function DA40_Flight_Model/Correlator Simulation/Subsystem1/Generating GPS and Satellite Measurements/Truth Model/Navigation1/DA-40 Equations of Motion/MATLAB Function4 ==
  data: m input; X_Dot output size=12; Ic_B input; F_B input; M_B input; X input; CG input; InvMassMatrix input
function X_Dot  = CalcXdot(m,Ic_B,F_B,M_B,X,CG,InvMassMatrix)
X_Dot = zeros(12,1);
% muVector = zeros(3,1);
u = X(1);
v = X(2);
w = X(3);
p = X(4);
q = X(5);
r = X(6);
x = X(7);
y = X(8);
z = X(9);
phi = X(10);
theta = X(11);
psi = X(12);


Xcg = CG(1);
Ycg = CG(2);
Zcg = CG(3);

CGssm = [0 -Zcg Ycg;Zcg 0 -Xcg;-Ycg Xcg 0];


lambdaX = F_B(1)/m + r*v - q*w - 0 - 2*q*0 + 2*r*0 + Xcg*(q^2 + r^2) - Ycg*p*q - Zcg*p*r;
lambdaY = F_B(2)/m + p*w - r*u - 0 - 2*r*0 + 2*p*0 - Xcg*p*q + Ycg*(p^2 +r^2) - Zcg*q*r;
lambdaZ = F_B(3)/m + q*u - p*v - 0 - 2*p*0 + 2*q*0 - Xcg*p*r - Ycg*q*r + Zcg*(p^2 + q^2);

MomentVector = [p;q;r];

MomentVectorssm = [0 -r q;r 0 -p;-q p 0];

muVector = [M_B(1);M_B(2);M_B(3)] - (MomentVectorssm*Ic_B*MomentVector) - m*CGssm*MomentVectorssm*[u;v;w];
LAMEparams = [lambdaX;lambdaY;lambdaZ;muVector];
X_Dot(1:6) = InvMassMatrix*LAMEparams;

cphi = cos(phi);
sphi = sin(phi);

ctheta = cos(theta);
stheta = sin(theta);
ttheta = tan(theta);

cpsi = cos(psi);
spsi = sin(psi);

xdot = ctheta*cpsi*u + sphi*stheta*cpsi - cphi*spsi*v + cphi*stheta*cpsi + sphi*spsi*w;
ydot = ctheta*spsi*u + sphi*stheta*spsi + cphi*cpsi*v + cphi*stheta*spsi - sphi*cpsi*w;
zdot = -stheta*u + sphi*ctheta*v + cphi*ctheta*w;
phidot = p + q*sphi*ttheta + r*cphi*ttheta;
thdot = q*cphi - r*sphi;
psidot = q*sphi/ctheta + r*cphi/ctheta;
X_Dot(7:12) = [xdot;ydot;zdot;phidot;thdot;psidot];

end

== matlab function DA40_Flight_Model/Extended Kalman Filter/Noise Model/Navigation/Flight Mechanics and Systems Models/Gravity/MATLAB Function ==
  data: X input; F_grav_b output; Mass_Properties input; CG input; M_grav_b output
function [F_grav_b,M_grav_b] = Grav_Forces(X,Mass_Properties,CG)
%% Defining State Vector to Code Easier
u = X(1);
v = X(2);
w = X(3);
p = X(4);
q = X(5);
r = X(6);
x = X(7);
y = X(8);
z = X(9);
phi = X(10);
theta = X(11);
psi = X(12);

g = 9.81;

F_grav_b = Mass_Properties.*[-g*sin(theta);g*sin(phi)*cos(theta);g*cos(phi)*cos(theta)];

M_grav_b = cross(CG,F_grav_b);

== matlab function DA40_Flight_Model/Extended Kalman Filter/Noise Model/Navigation/Flight Mechanics and Systems Models/Strip Theory Aero + Propulsive Forces/Strip_Theory_Modeling ==
  data: atmos input; X input; U input; stripGeom input; Strip_Theory_Forces output; Strip_Theory_Moments output
function [Strip_Theory_Forces,Strip_Theory_Moments] = Strip_Theory(atmos,X,U,stripGeom)
Strip_Theory_Forces = [0;0;0];
Strip_Theory_Moments = [0;0;0];

coder.extrinsic('griddedInterpolant')
coder.extrinsic('AC_Strip_Theory')

[Strip_Theory_Forces,Strip_Theory_Moments] = AC_Strip_Theory(atmos(4),X,U,stripGeom);

== matlab function DA40_Flight_Model/Correlator Simulation/Subsystem1/Subsystem2/Subsystem3/Subsystem2/MATLAB Function1 ==
  data: samplesPerPDI input; initialCodeFrequency input; initialCodePhase input; codeChangePerSample output; measuredCodeFrequency input; initialCodePhase output; chipRate input; dSvClk input
function [codeChangePerSample,initialCodePhase]  = fcn(samplesPerPDI,initialCodeFrequency,initialCodePhase,measuredCodeFrequency,chipRate,dSvClk)

codeChangePerSample = (measuredCodeFrequency - initialCodeFrequency + dSvClk*chipRate)/samplesPerPDI;

initialCodePhase = initialCodePhase;

end

== matlab function DA40_Flight_Model/Correlator Simulation/Subsystem1/Subsystem2/Subsystem3/MATLAB Function1 ==
  data: svClockBias input; dSvClk output; initialSVClockBias input
function dSvClk = calculateClockDifference(svClockBias,initialSVClockBias)

dSvClk = svClockBias - initialSVClockBias;

end

== matlab function DA40_Flight_Model/Correlator Simulation/Subsystem1/Subsystem2/Subsystem3/MATLAB Function2 ==
  data: doppler input; measuredCodeFrequency output; chiprate input; L1freq input
function measuredCodeFrequency = fcn(doppler,chiprate,L1freq)

measuredCodeFrequency = doppler + chiprate/L1freq + chiprate;

== matlab function DA40_Flight_Model/Correlator Simulation/Subsystem1/Subsystem2/Subsystem3/MATLAB Function3 ==
  data: initialDoppler input; initialCodeFrequency output; initialChiprate input; L1freq input
function initialCodeFrequency = fcn(initialDoppler,initialChiprate,L1freq)

initialCodeFrequency = initialDoppler + initialChiprate/L1freq + initialChiprate;

== matlab function DA40_Flight_Model/Correlator Simulation/Subsystem1/Generating GPS and Satellite Measurements1/Body To ECEF/MATLAB Function1 ==
  data: x output; pos input; y output; vel input; clk input; clkBias input; DCM_BL input; z output; u output; v output; w output; clk output; clkBias output; refLL input
function [x,y,z,u,v,w,clk,clkBias] = BodyToEarthStates(pos,vel,clk,clkBias,DCM_BL,refLL)
x = 0;
y = 0;
z = 0;
u = 0;
v = 0;
w = 0;

coder.extrinsic("BodyToEarthStates")

[x,y,z,u,v,w,clk,clkBias] = BodyToEarthStates(pos,vel,clk,clkBias,DCM_BL,refLL);

end

== matlab function DA40_Flight_Model/Correlator Simulation/Subsystem1/Generating GPS and Satellite Measurements1/Calculate Satellite Positions/MATLAB Function ==
  data: transmitTime input; satelliteID input; toe input; a_f2 input; a_f1 input; a_f0 input; T_GD input; sqrtA input; Eccentricity input; C_us input; C_uc input; satX output; satY output; satZ output; satU output; satV output; satW output; satClkCorr output; C_rs input; C_rc input; C_is input; C_ic input; M_0 input; iDOT input; i_0 input; OMEGA input; OMEGA_DOT input; delta_n input; OMEGA_0 input
function [satX,satY,satZ,satU,satV,satW,satClkCorr] = satpos(transmitTime,satelliteID,toe,a_f2,a_f1,a_f0,T_GD,sqrtA,Eccentricity,C_us,C_uc,C_rs,C_rc,C_is,C_ic,M_0,iDOT,i_0,OMEGA,OMEGA_DOT,delta_n,OMEGA_0)

%% Initialize constants ===================================================
numOfSatellites = length(satelliteID);

% GPS constatns

gpsPi          = 3.1415926535898;  % Pi used in the GPS coordinate
% system

%--- Constants for satellite position calculation -------------------------
Omegae_dot     = 7.2921151467e-5;  % Earth rotation rate, [rad/s]
GM             = 3.986005e14;      % Earth's universal
% gravitational parameter,
% [m^3/s^2]
F              = -4.442807633e-10; % Constant, [sec/(meter)^(1/2)]

%% Initialize results =====================================================
satClkCorr   = zeros(1,numOfSatellites);
satX = zeros(1,numOfSatellites);
satY = zeros(1,numOfSatellites);
satZ = zeros(1,numOfSatellites);
satU = zeros(1,numOfSatellites);
satV = zeros(1,numOfSatellites);
satW = zeros(1,numOfSatellites);

%% Process each satellite =================================================

for satNr = 1 : numOfSatellites

    %% Find initial satellite clock correction --------------------------------

    %--- Find time difference ---------------------------------------------
    dt = check_t(transmitTime(satNr) - toe(satNr));

    %--- Calculate clock correction ---------------------------------------
    satClkCorr(satNr) = (a_f2(satNr) * dt + a_f1(satNr)) * dt + ...
        a_f0(satNr) - ...
        T_GD(satNr);
    time = transmitTime(satNr) - satClkCorr(satNr);

    %% Find satellite's position ----------------------------------------------

    % Restore semi-major axis
    a   = sqrtA(satNr)*sqrtA(satNr);

    % Time correction
    tk  = check_t(time - toe(satNr));

    % Initial mean motion
    n0  = sqrt(GM/a^3);
    % Mean motion
    n   = n0 + delta_n(satNr);

    % Mean anomaly
    M   = M_0(satNr) + n*tk;
    % Reduce mean anomaly to between 0 and 360 deg
    M   = rem(M + 2*gpsPi, 2*gpsPi);

    % Initial guess of eccentric anomaly
    E   = M;

    %--- Iteratively compute eccentric anomaly ----------------------------
    for ii = 1:10
        E_old   = E;
        E       = M + Eccentricity(satNr) * sin(E);
        dE      = rem(E - E_old, 2*gpsPi);

        if abs(dE) < 1.e-12
            % Necessary precision is reached, exit from the loop
            break;
        end
    end

    % Reduce eccentric anomaly to between 0 and 360 deg
    E   = rem(E + 2*gpsPi, 2*gpsPi);
    dE = n/(1-Eccentricity(satNr) * cos(E));
    % Compute relativistic correction term
    dtr = F * Eccentricity(satNr) * sqrtA(satNr) * sin(E);

    % Calculate the true anomaly
    nu   = atan2(sqrt(1 - Eccentricity(satNr)^2) * sin(E), cos(E)-Eccentricity(satNr));

    %Compute angle phi
    phi = nu + OMEGA(satNr);
    dphi=sqrt(1-Eccentricity(satNr)^2)*dE/(1-Eccentricity(satNr)*cos(E));
    % Reduce phi to between 0 and 360 deg
    phi = rem(phi, 2*gpsPi);

    % Correct argument of latitude
    u = phi + ...
        C_uc(satNr) * cos(2*phi) + ...
        C_us(satNr) * sin(2*phi);
    du=(1+2*(C_us(satNr) * cos(2*phi)-C_uc(satNr) * sin(2*phi)))*dphi;
    % Correct radius
    r = a * (1 - Eccentricity(satNr)*cos(E)) + ...
        C_rc(satNr) * cos(2*phi) + ...
        C_rs(satNr) * sin(2*phi);
    dr= a * Eccentricity(satNr) *sin(E) *dE + ...
        2 * (C_rs(satNr) * cos(2*phi) - C_rc(satNr) * sin(2*phi)) ...
        * dphi;
    % Correct inclination
    i = i_0(satNr) + iDOT(satNr) * tk + ...
        C_ic(satNr) * cos(2*phi) + ...
        C_is(satNr) * sin(2*phi);
    di = 2 * (C_is(satNr) * cos(2*phi) - C_ic(satNr) * sin(2*phi)) ...
        * dphi + iDOT(satNr);

    % Compute the angle between the ascending node and the Greenwich meridian
    Omega = OMEGA_0(satNr) + (OMEGA_DOT(satNr) - Omegae_dot)*tk - ...
        Omegae_dot * toe(satNr);
    dOmega = OMEGA_DOT(satNr) - Omegae_dot;
    % Reduce to between 0 and 360 deg
    Omega = rem(Omega + 2*gpsPi, 2*gpsPi);

    %--- Compute satellite coordinates ------------------------------------
    x = cos(u)*r * cos(Omega) - sin(u)*r * cos(i)*sin(Omega);
    y = cos(u)*r * sin(Omega) + sin(u)*r * cos(i)*cos(Omega);
    z = sin(u)*r * sin(i);

    xdash = r * cos(u);
    ydash = r * sin(u);

    dxdash = dr * cos(u) - r * sin(u) * du;
    dydash = dr * sin(u) + r * cos(u) * du;

    Vx = dxdash * cos(Omega) -  dydash * cos(i) * sin(Omega) ...
        + ydash * sin(Omega) * sin(i) * di - (xdash * sin(Omega) + ...
        ydash * cos(i) * cos(Omega)) * dOmega;

    Vy = dxdash * sin(Omega) + dydash * cos(i) * cos(Omega) - ...
        ydash * sin(i) *cos(Omega) * di + (xdash * cos(Omega) - ...
        ydash * cos(i) * sin(Omega)) * dOmega;

    Vz = dydash * sin(i) + ydash * cos(i) * di;

    satX(satNr) = x;
    satY(satNr) = y;
    satZ(satNr) = z;
    satU(satNr) = Vx;
    satV(satNr) = Vy;
    satW(satNr) = Vz;

    % Include relativistic correction in clock correction --------------------
    satClkCorr(satNr) = (a_f2(satNr) * dt + a_f1(satNr)) * dt + ...
        a_f0(satNr) - ...
        T_GD(satNr) + dtr;

end % for satNr = 1 : numOfSatellites

end

function corrTime = check_t(time)

%CHECKTIME is a subfunction of SATPOS used to check for
%overlapping time in GPS seconds

half_week = 302400;     % seconds

corrTime = time;

if time > half_week
    corrTime = time - 2*half_week;
elseif time < -half_week
    corrTime = time + 2*half_week;
end
end

== matlab function DA40_Flight_Model/Correlator Simulation/Subsystem1/Generating GPS and Satellite Measurements1/Truth Model/Control/Subsystem3/MATLAB Function ==
  data: X input; Aircraft_Airspeed output
function Aircraft_Airspeed = Calc_AC_Speed(X)
Aircraft_Airspeed = norm(X(1:3));
end

== matlab function DA40_Flight_Model/Correlator Simulation/Subsystem1/Generating GPS and Satellite Measurements1/Truth Model/Environment/MATLAB Function ==
  data: windVectorNav input; windVectorBody output; states input
function windVectorBody = windRotation(windVectorNav,states)

DCMBN = genDCM('rad',[states(12),states(11),states(10)], [3 2 1]);

windVectorBody = DCMBN'*[windVectorNav; 0];

end

== matlab function DA40_Flight_Model/Correlator Simulation/Subsystem1/Generating GPS and Satellite Measurements/Truth Model/Guidance/MATLAB Function ==
  data: heading input; heading output
function heading = fcn(heading)

heading = wrapTo360(heading*180/pi);

end

== matlab function DA40_Flight_Model/Correlator Simulation/Subsystem1/Generating GPS and Satellite Measurements1/Truth Model/Guidance/MATLAB Function ==
  data: heading input; heading output
function heading = fcn(heading)

heading = wrapTo360(heading*180/pi);

end

== matlab function DA40_Flight_Model/Correlator Simulation/Subsystem1/Generating GPS and Satellite Measurements1/Truth Model/Navigation1/DA-40 Equations of Motion/MATLAB Function4 ==
  data: m input; X_Dot output size=12; Ic_B input; F_B input; M_B input; X input; CG input; InvMassMatrix input
function X_Dot  = CalcXdot(m,Ic_B,F_B,M_B,X,CG,InvMassMatrix)
X_Dot = zeros(12,1);
% muVector = zeros(3,1);
u = X(1);
v = X(2);
w = X(3);
p = X(4);
q = X(5);
r = X(6);
x = X(7);
y = X(8);
z = X(9);
phi = X(10);
theta = X(11);
psi = X(12);


Xcg = CG(1);
Ycg = CG(2);
Zcg = CG(3);

CGssm = [0 -Zcg Ycg;Zcg 0 -Xcg;-Ycg Xcg 0];


lambdaX = F_B(1)/m + r*v - q*w - 0 - 2*q*0 + 2*r*0 + Xcg*(q^2 + r^2) - Ycg*p*q - Zcg*p*r;
lambdaY = F_B(2)/m + p*w - r*u - 0 - 2*r*0 + 2*p*0 - Xcg*p*q + Ycg*(p^2 +r^2) - Zcg*q*r;
lambdaZ = F_B(3)/m + q*u - p*v - 0 - 2*p*0 + 2*q*0 - Xcg*p*r - Ycg*q*r + Zcg*(p^2 + q^2);

MomentVector = [p;q;r];

MomentVectorssm = [0 -r q;r 0 -p;-q p 0];

muVector = [M_B(1);M_B(2);M_B(3)] - (MomentVectorssm*Ic_B*MomentVector) - m*CGssm*MomentVectorssm*[u;v;w];
LAMEparams = [lambdaX;lambdaY;lambdaZ;muVector];
X_Dot(1:6) = InvMassMatrix*LAMEparams;

cphi = cos(phi);
sphi = sin(phi);

ctheta = cos(theta);
stheta = sin(theta);
ttheta = tan(theta);

cpsi = cos(psi);
spsi = sin(psi);

xdot = ctheta*cpsi*u + sphi*stheta*cpsi - cphi*spsi*v + cphi*stheta*cpsi + sphi*spsi*w;
ydot = ctheta*spsi*u + sphi*stheta*spsi + cphi*cpsi*v + cphi*stheta*spsi - sphi*cpsi*w;
zdot = -stheta*u + sphi*ctheta*v + cphi*ctheta*w;
phidot = p + q*sphi*ttheta + r*cphi*ttheta;
thdot = q*cphi - r*sphi;
psidot = q*sphi/ctheta + r*cphi/ctheta;
X_Dot(7:12) = [xdot;ydot;zdot;phidot;thdot;psidot];

end

== matlab function DA40_Flight_Model/Correlator Simulation/Subsystem1/Generating GPS and Satellite Measurements1/Truth Model/Navigation1/Flight Mechanics and Systems Models/Engine + Prop Model/Subsystem/Air Flow Rate Exam 1 ==
  data: Tatm_K input; Pman_inHg input; throttle input; Patm_inHg input; Air_lb_hr output
function Air_lb_hr  = Calc_Air_Flow(Tatm_K,Pman_inHg,throttle,Patm_inHg)
%% Conversion Factors
inHg_to_Pa = 3386.39;
in2_to_m2 = 0.00064516;
kg_to_lb = 2.20462;
%% Constants
gamma = 1.4;
R = 287;
AirflowScaler = 0.69 * 0.95;
DischargeCoeff = 0.6;
th = 70*throttle;
D = 2.75;

Patm_Pa = Patm_inHg * inHg_to_Pa;
Pman_Pa = Pman_inHg * inHg_to_Pa;
A_in2 = (pi/4) * D^2 *  (0.01 + (1-0.01)*(1 - cosd(th)));
A_m2 = A_in2 * in2_to_m2;

Threshold_X = (2/(gamma+1))^(gamma/(gamma-1));

x = Threshold_X;

MAF = sqrt((2*gamma/(gamma-1))*(x^(2/gamma)-x^((gamma+1)/gamma)));

MassFlux_kgm2s = MAF*Patm_Pa/sqrt(R*Tatm_K);
MassFlow_kgs = MassFlux_kgm2s * A_m2; 

Air_lb_hr = AirflowScaler*DischargeCoeff*MassFlow_kgs*3600*kg_to_lb;
end

== matlab function DA40_Flight_Model/Correlator Simulation/Subsystem1/Generating GPS and Satellite Measurements1/Truth Model/Navigation1/Flight Mechanics and Systems Models/Engine + Prop Model/Subsystem/Engine Shaft Power and Torque Model ==
  data: wdot_f input; PF input; BSFC input; P_shaft output
function P_shaft  = fcn(wdot_f,PF,BSFC)

P_shaft = PF*wdot_f/BSFC; %hp

% Q_drive = P_shaft*746/Omega; %Nm


end
